simulink model "position_control_2015"  (R2020a)
settings: Solver=ode4  StartTime=0.0  StopTime=inf  FixedStep=0.002  RelTol=1e-3  EnableMultiTasking=on
undefined symbols (not defined in the file): Afe, g, gain_stab9, gains_increasing, I_eq_increasing, K, Kp_i_increasing, Kp_mf_increasing, L, m, m0, REG_m9_f, Ti_i_increasing, Ti_mf_increasing, x, x_eq, x_eq_increasing, y
libraries: simulink x8, PoliArd x6
settings Model: ExtModeTrigDuration=2  Creator=User  LastModifiedBy=miche
settings DataIOCC: LimitDataPoints=on  SaveFormat=Array  ReturnWorkspaceOutputs=off
settings OptimizationCC: LifeSpan=1  EfficientTunableParamExpr=on
settings DebuggingCC: UnderspecifiedInitializationDetection=Classic  MergeDetectMultiDrivingBlocksExec=none  SFUnexpectedBacktrackingDiag=warning  SFNoUnconditionalDefaultTransitionDiag=warning  SFExecutionAtInitializationDiag=none  ArithmeticOperatorsInVariantConditions=warning
settings HardwareCC: ProdBitPerPointer=32  ProdBitPerSizeT=32  ProdBitPerPtrDiffT=32  ProdLargestAtomicInteger=Long  ProdLargestAtomicFloat=Double  ProdIntDivRoundTo=Undefined  ProdWordSize=32  ProdHWDeviceType=ARM Compatible->ARM Cortex
settings ModelReferenceCC: PropagateSignalLabelsOutOfModel=off
settings SFSimCC: SimUseLocalCustomCode=off  MATLABDynamicMemAlloc=off  CustomCodeUndefinedFunction=UseInterfaceOnly
settings RTWCC: Description=Run on Target Hardware  SystemTargetFile=realtime.tlc  GenerateMakefile=off  TemplateMakefile=realtime.tmf  RTWVerbose=off  RTWUseLocalCustomCode=off
settings CodeAppCC: StateflowObjectComments=on
settings STFCustomTargetCC: TargetLibSuffix=.a  GenerateSampleERTMain=on  ERTCustomFileBanners=on  SupportNonInlinedSFcns=off  RemoveResetFunc=on  SupportVariableSizeSignals=on  MATLABClassNameForMDSCustomization=Simulink.SoftwareTarget.ERTCustomization  SystemTargetFile=realtime.tlc
settings ERTTargetCC: MultiwordLength=2048  GenerateSampleERTMain=on  ParMdlRefBuildCompliant=off  CompOptLevelCompliant=off  ConcurrentExecutionCompliant=off  CombineOutputUpdateFcns=off  SupportContinuousTime=on  SupportVariableSizeSignals=on  ModelStepFunctionPrototypeControlCompliant=off  CPPClassGenCompliant=off  UseToolchainInfoCompliant=off  ExtModeTransport=3  ExtModeMexFile=ext_serial_win32_comm_rtt  ExtModeMexArgs=0 1 9600  ERTSrcFileBannerTemplate=realtime_code_template.cgt  ERTHdrFileBannerTemplate=realtime_code_template.cgt  ERTDataSrcFileTemplate=realtime_code_template.cgt  ERTDataHdrFileTemplate=realtime_code_template.cgt  ERTCustomFileTemplate=realtime_file_process.tlc  ConvertIfToSwitch=off  SuppressUnreachableDefaultCases=off
settings ConfigComp: CovMetricSettings=dw  CovSaveCumulativeToWorkspaceVar=on  CovSaveSingleToWorkspaceVar=on  CovExternalEMLEnable=off

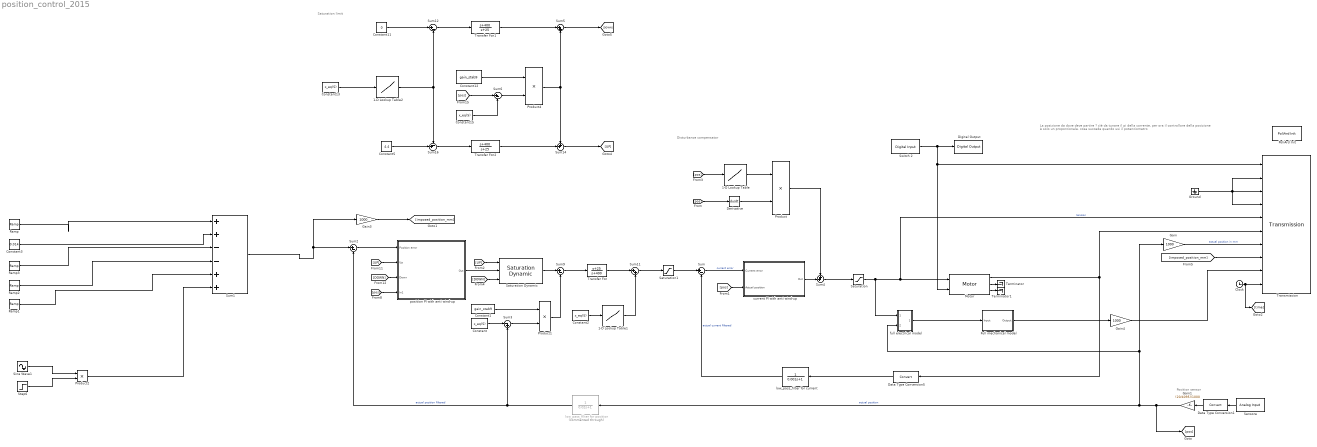
== system position_control_2015 ==
  note: Saturation limit
  note: Position sensor
  note: Disturbance compensator
  note: La posizione da dove deve partire ? cìè da tunare il pi della corrente, per ora il controllore della posizione è solo un
      | proporzionale. cosa succede quando usi il potenziometro
  1-D Lookup Table : Lookup_n-D  NumberOfTableDimensions=1  BreakpointsForDimension1=[0.0085 x_eq_increasing]  Table=[gains_increasing(1) gains_increasing]  InternalRulePriority=Speed  RndMeth=Simplest  InputSameDT=on
  1-D Lookup Table1 : Lookup_n-D  NumberOfTableDimensions=1  BreakpointsForDimension1=[0.0085 x_eq_increasing]  Table=[3.55 I_eq_increasing]  InternalRulePriority=Speed  RndMeth=Simplest  InputSameDT=on
  1-D Lookup Table2 : Lookup_n-D  NumberOfTableDimensions=1  BreakpointsForDimension1=[0.0085 x_eq_increasing]  Table="[3.55  I_eq_increasing]"  InternalRulePriority=Speed  RndMeth=Simplest  InputSameDT=on
  Clock : Clock
  Constant{,2,13,15} (4 alike) : Constant  Value=x_eq(5)
  Constant1 : Constant  Value=gain_stab9
  Constant11 : Constant  Value=0
  Constant12 : Constant  Value=gain_stab9
  Constant3 : Constant  Value=0.014
  Constant5 : Constant  Value=4.4
  Data Type Conversion1 : DataTypeConversion
  Data Type Conversion5 : DataTypeConversion
  Derivative : Derivative
  Digital Output : PoliArd/Digital Output  DO_pin=1
  Full mechanical model : Subsystem
  Gain : Gain  Gain=1000
  Gain1 : Gain  Gain=(20/4095)/1000
  Gain3 : Gain  Gain=1000
  Gain4 : Gain  Gain=1000
  Ground : Ground
  Motor : PoliArd/Motor  MotorID=2  DC_bus_mask=24  dt_mot=-1
  PoliArd Init : PoliArd/PoliArd Init
  Product{,1..2,4} (4 alike) : Product
  Ramp : simulink/Sources/Ramp  slope=0.001  start=7  InitialOutput=0
  Ramp1 : simulink/Sources/Ramp  slope=0.001  start=19  InitialOutput=0
  Ramp2 : simulink/Sources/Ramp  slope=0.001  start=17  InitialOutput=0
  Ramp3 : simulink/Sources/Ramp  slope=0.001  start=12  InitialOutput=0
  Saturation : Saturate  UpperLimit=18  LowerLimit=0
  Saturation Dynamic : simulink/Discontinuities/Saturation Dynamic  OutMin=[]  OutMax=[]  OutDataTypeStr=Inherit: Same as second input  OutDataType=fixdt(1, 16)  OutScaling=2^-10  DoSatur=off
  Saturation1 : Saturate  UpperLimit=4.4  LowerLimit=0
  Sensore : PoliArd/Analog Input  AIpin_mask=2  AIsample=-1
  Sine Wave1 : Sin  Amplitude=0.002  Phase=0.3  SampleTime=0
  Step6 : Step  Time=28  SampleTime=0
  Sum{,2,6,9,12} (5 alike) : Sum  Inputs=|+-
  Sum1 : Sum  Inputs=|++--++
  Sum11 : Sum  Inputs=|++
  Sum14 : Sum  Inputs=++|
  Sum16 : Sum  Inputs=-+|
  Sum3 : Sum  Inputs=|-+
  Sum4 : Sum  Inputs=++|
  Sum5 : Sum  Inputs=|++
  Switch 2 : PoliArd/Digital Input  DI_pin=2  DIsample=-1
  Terminator : Terminator
  Terminator1 : Terminator
  Transfer Fcn : TransferFcn  Numerator=[1 25]  Denominator=[1 400]
  Transfer Fcn1 : TransferFcn  Numerator=[1 400]  Denominator=[1 25]
  Transfer Fcn2 : TransferFcn  Numerator=[1 400]  Denominator=[1 25]
  Transmission : PoliArd/Transmission  sample_freq=500  sig_to_send=6
  current PI with anti wind-up : Subsystem
      mask Display: disp('Current controller\n(PI)\nwith anti wind-up')
  full electrical model : Subsystem
  low_pass_filter for current : TransferFcn  Denominator=[0.001 1]
  low_pass_filter for position : TransferFcn  Commented=through  Denominator=[0.02 1]
  position PI with anti wind-up : Subsystem
      mask Display: disp('Position controller\n(PI)\nwith anti wind-up')
  wires:
  Switch 2/1 -> Digital Output/1, Motor/2, Transmission/1
  Sensore/1 -> Data Type Conversion1/1
  Ground/1 -> Transmission/2, Transmission/4, Transmission/3
  Motor/1 -> Data Type Conversion5/1, Transmission/6
  Data Type Conversion1/1 -> Gain1/1
  Saturation/1 -> full electrical model/1(In1), Transmission/5, Motor/1  "tension"
  Constant1/1 -> Product1/1
  Sum9/1 -> Transfer Fcn/1
  Sum11/1 -> Saturation1/1
  [DOWN] -> Saturation Dynamic/3
  1-D Lookup Table1/1 -> Sum11/2
  Product/1 -> Sum4/1
  Saturation Dynamic/1 -> Sum9/1
  Derivative/1 -> Product/2
  Sum2/1 -> position PI with anti wind-up/1(Position error)
  1-D Lookup Table/1 -> Product/1
  current PI with anti wind-up/1(Out) -> Sum4/2
  Sum/1 -> current PI with anti wind-up/1(Current error)  "current error"
  position PI with anti wind-up/1(Out) -> Saturation Dynamic/2
  [pos] -> 1-D Lookup Table/1
  Sum3/1 -> Product1/2
  Product1/1 -> Sum9/2
  [UP] -> Saturation Dynamic/1
  Transfer Fcn/1 -> Sum11/1
  [pos] -> current PI with anti wind-up/2(Actual position)
  Sum4/1 -> Saturation/1
  Saturation1/1 -> Sum/1
  [pos] -> Derivative/1
  Data Type Conversion5/1 -> low_pass_filter for current/1
  Gain1/1 -> full electrical model/2(In2), Gain/1, low_pass_filter for position/1, [pos]  "actual position"
  low_pass_filter for current/1 -> Sum/2  "actual current filtered"
  low_pass_filter for position/1 -> Sum2/2, Sum3/2  "actual position filtered"
  Constant2/1 -> 1-D Lookup Table1/1
  Gain/1 -> Transmission/7  "actual position in mm"
  [DOWN] -> position PI with anti wind-up/3(Down)
  [UP] -> position PI with anti wind-up/2(Up)
  [imposed_position_mm] -> Transmission/8
  Motor/2 -> Terminator/1
  Motor/3 -> Terminator1/1
  Constant/1 -> Sum3/1
  Sum5/1 -> [DOWN]
  Constant15/1 -> Sum6/2
  Sum12/1 -> Transfer Fcn1/1
  Product4/1 -> Sum14/1, Sum5/2
  1-D Lookup Table2/1 -> Sum16/1, Sum12/2
  Sum16/1 -> Transfer Fcn2/1
  Sum6/1 -> Product4/2
  Constant13/1 -> 1-D Lookup Table2/1
  Constant11/1 -> Sum12/1
  [pos] -> Sum6/1
  Transfer Fcn2/1 -> Sum14/2
  Sum14/1 -> [UP]
  Transfer Fcn1/1 -> Sum5/1
  Constant12/1 -> Product4/1
  Constant5/1 -> Sum16/2
  [pos] -> position PI with anti wind-up/4(In1)
  Gain3/1 -> [imposed_position_mm]
  Clock/1 -> Transmission/10, [time]
  Ramp/1 -> Sum1/1
  Constant3/1 -> Sum1/2
  Ramp3/1 -> Sum1/3
  Ramp2/1 -> Sum1/4
  Ramp1/1 -> Sum1/5
  Sine Wave1/1 -> Product2/1
  Step6/1 -> Product2/2
  Product2/1 -> Sum1/6
  Sum1/1 -> Gain3/1, Sum2/1
  full electrical model/1(Input) -> Full mechanical model/1(Input)
  Full mechanical model/1(Output) -> Gain4/1
  Gain4/1 -> Transmission/9

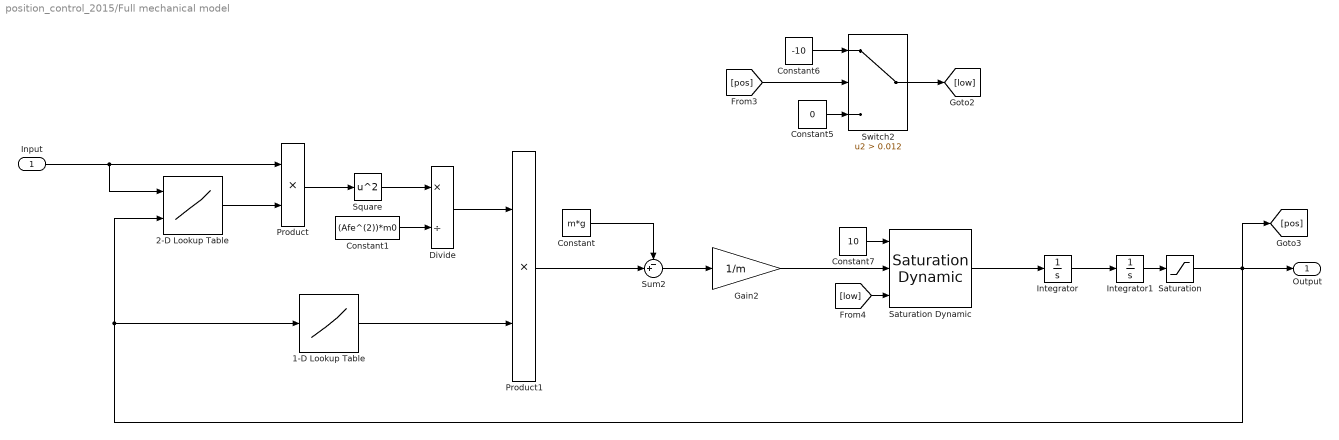
== system position_control_2015/Full mechanical model ==
  Input : Inport
  1-D Lookup Table : Lookup_n-D  NumberOfTableDimensions=1  BreakpointsForDimension1=x  Table=K  InternalRulePriority=Speed  RndMeth=Simplest  InputSameDT=on
  2-D Lookup Table : Lookup_n-D  BreakpointsForDimension1=y  BreakpointsForDimension2=x  Table=L  InternalRulePriority=Speed  RndMeth=Simplest  InputSameDT=on
  Constant : Constant  Value=m*g
  Constant1 : Constant  Value=(Afe^(2))*m0
  Constant5 : Constant  Value=0
  Constant6 : Constant  Value=-10
  Constant7 : Constant  Value=10
  Divide : Product  Inputs=*/
  Gain2 : Gain  Gain=1/m
  Integrator : Integrator
  Integrator1 : Integrator  InitialCondition=0.0085
  Product : Product
  Product1 : Product
  Saturation : Saturate  UpperLimit=0.020  LowerLimit=0.0085
  Saturation Dynamic : simulink/Discontinuities/Saturation Dynamic  OutMin=[]  OutMax=[]  OutDataTypeStr=Inherit: Same as second input  OutDataType=fixdt(1, 16)  OutScaling=2^-10  DoSatur=off
  Square : Math  Operator=square  SignedPower=on  SaturateOnIntegerOverflow=on
  Sum2 : Sum  Inputs=-+|
  Switch2 : Switch  Criteria=u2 > Threshold  Threshold=0.012
  Output : Outport
  wires:
  Input/1 -> Product/1, 2-D Lookup Table/1
  Square/1 -> Divide/1
  Constant/1 -> Sum2/1
  Product1/1 -> Sum2/2
  Product/1 -> Square/1
  Constant1/1 -> Divide/2
  2-D Lookup Table/1 -> Product/2
  Divide/1 -> Product1/1
  1-D Lookup Table/1 -> Product1/2
  Integrator1/1 -> Saturation/1
  Integrator/1 -> Integrator1/1
  Sum2/1 -> Gain2/1
  Constant6/1 -> Switch2/1
  [pos] -> Switch2/2
  Switch2/1 -> [low]
  Constant5/1 -> Switch2/3
  [low] -> Saturation Dynamic/3
  Constant7/1 -> Saturation Dynamic/1
  Saturation/1 -> 1-D Lookup Table/1, 2-D Lookup Table/2, Output/1, [pos]
  Gain2/1 -> Saturation Dynamic/2
  Saturation Dynamic/1 -> Integrator/1

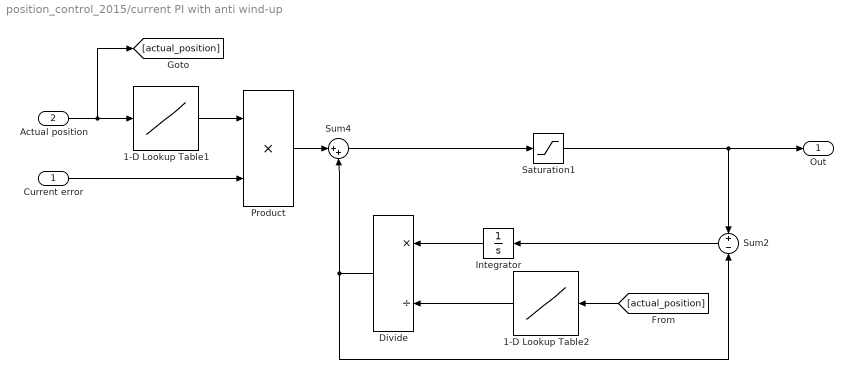
== system position_control_2015/current PI with anti wind-up ==
  Current error : Inport
  Actual position : Inport  Port=2
  1-D Lookup Table1 : Lookup_n-D  NumberOfTableDimensions=1  BreakpointsForDimension1=[0.0085 x_eq_increasing]  Table=[Kp_i_increasing(1) Kp_i_increasing]  InternalRulePriority=Speed  RndMeth=Simplest  InputSameDT=on
  1-D Lookup Table2 : Lookup_n-D  NumberOfTableDimensions=1  BreakpointsForDimension1=[0.0085 x_eq_increasing]  Table=[Ti_i_increasing(1) Ti_i_increasing]  InternalRulePriority=Speed  RndMeth=Simplest  InputSameDT=on
  Divide : Product  Inputs=*/
  Integrator : Integrator
  Product : Product
  Saturation1 : Saturate  UpperLimit=18  LowerLimit=0
  Sum2 : Sum  Inputs=+|-
  Sum4 : Sum  Inputs=|++
  Out : Outport
  wires:
  Sum4/1 -> Saturation1/1
  Product/1 -> Sum4/1
  Saturation1/1 -> Out/1, Sum2/1
  Current error/1 -> Product/2
  1-D Lookup Table1/1 -> Product/1
  Actual position/1 -> [actual_position], 1-D Lookup Table1/1
  Divide/1 -> Sum2/2, Sum4/2
  Sum2/1 -> Integrator/1
  Integrator/1 -> Divide/1
  1-D Lookup Table2/1 -> Divide/2
  [actual_position] -> 1-D Lookup Table2/1

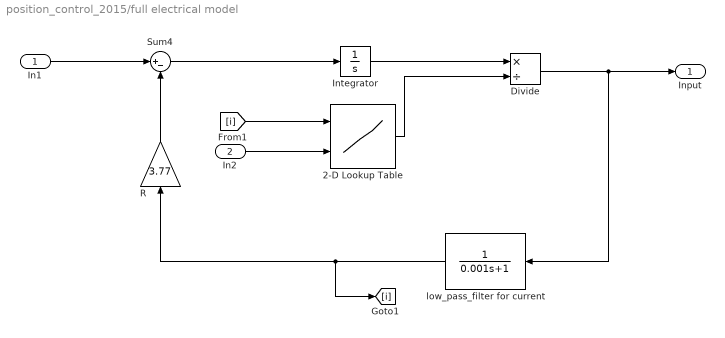
== system position_control_2015/full electrical model ==
  In1 : Inport
  In2 : Inport  Port=2
  2-D Lookup Table : Lookup_n-D  BreakpointsForDimension1=y  BreakpointsForDimension2=x  Table=L  InternalRulePriority=Speed  RndMeth=Simplest  InputSameDT=on
  Divide : Product  Inputs=*/
  Integrator : Integrator
  R : Gain  Gain=3.77
  Sum4 : Sum  Inputs=|+-
  low_pass_filter for current : TransferFcn  Denominator=[0.001 1]
  Input : Outport
  wires:
  Sum4/1 -> Integrator/1
  Integrator/1 -> Divide/1
  R/1 -> Sum4/2
  In2/1 -> 2-D Lookup Table/2
  2-D Lookup Table/1 -> Divide/2
  In1/1 -> Sum4/1
  [i] -> 2-D Lookup Table/1
  Divide/1 -> low_pass_filter for current/1, Input/1
  low_pass_filter for current/1 -> [i], R/1

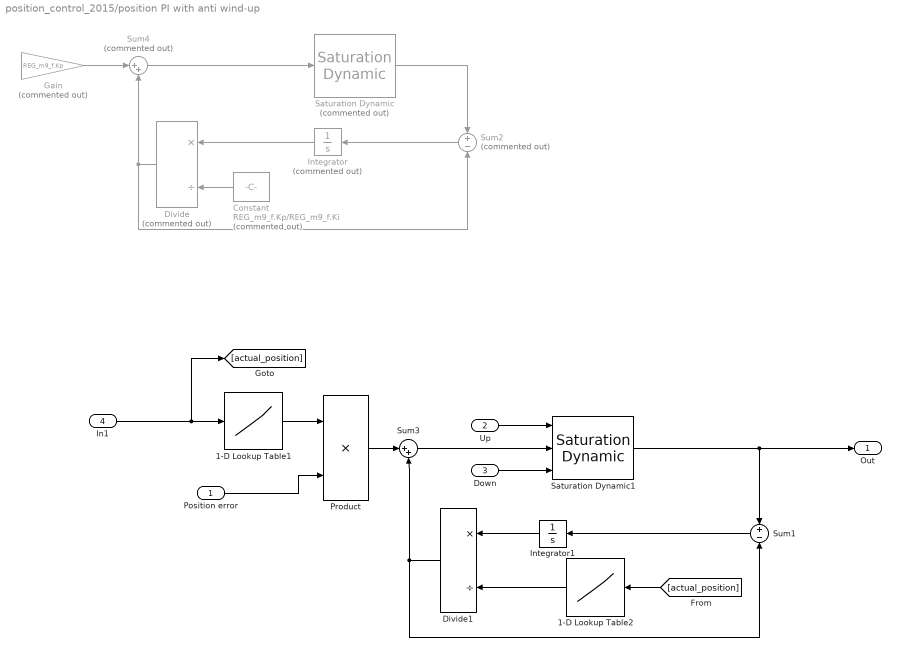
== system position_control_2015/position PI with anti wind-up ==
  Position error : Inport
  Up : Inport  Port=2
  Down : Inport  Port=3
  In1 : Inport  Port=4
  1-D Lookup Table1 : Lookup_n-D  NumberOfTableDimensions=1  BreakpointsForDimension1=[0.0085 x_eq_increasing]  Table=[Kp_mf_increasing(1) Kp_mf_increasing]  InternalRulePriority=Speed  RndMeth=Simplest  InputSameDT=on
  1-D Lookup Table2 : Lookup_n-D  NumberOfTableDimensions=1  BreakpointsForDimension1=[0.0085 x_eq_increasing]  Table=[Ti_mf_increasing(1) Ti_mf_increasing]  InternalRulePriority=Speed  RndMeth=Simplest  InputSameDT=on
  Constant : Constant  Commented=on  Value=REG_m9_f.Kp/REG_m9_f.Ki
  Divide : Product  Commented=on  Inputs=*/
  Divide1 : Product  Inputs=*/
  Gain : Gain  Commented=on  Gain=REG_m9_f.Kp
  Integrator : Integrator  Commented=on
  Integrator1 : Integrator
  Product : Product
  Saturation Dynamic : simulink/Discontinuities/Saturation Dynamic  Commented=on  OutMin=[]  OutMax=[]  OutDataTypeStr=Inherit: Same as second input  OutDataType=fixdt(1, 16)  OutScaling=2^-10  DoSatur=off
  Saturation Dynamic1 : simulink/Discontinuities/Saturation Dynamic  OutMin=[]  OutMax=[]  OutDataTypeStr=Inherit: Same as second input  OutDataType=fixdt(1, 16)  OutScaling=2^-10  DoSatur=off
  Sum1 : Sum  Inputs=+|-
  Sum2 : Sum  Commented=on  Inputs=+|-
  Sum3 : Sum  Inputs=|++
  Sum4 : Sum  Commented=on  Inputs=|++
  Out : Outport
  wires:
  Gain/1 -> Sum4/1
  Constant/1 -> Divide/2
  Sum2/1 -> Integrator/1
  Divide/1 -> Sum2/2, Sum4/2
  Integrator/1 -> Divide/1
  Sum4/1 -> Saturation Dynamic/2
  Saturation Dynamic/1 -> Sum2/1
  [actual_position] -> 1-D Lookup Table2/1
  Divide1/1 -> Sum1/2, Sum3/2
  1-D Lookup Table2/1 -> Divide1/2
  Integrator1/1 -> Divide1/1
  Sum1/1 -> Integrator1/1
  1-D Lookup Table1/1 -> Product/1
  Saturation Dynamic1/1 -> Out/1, Sum1/1
  Product/1 -> Sum3/1
  Sum3/1 -> Saturation Dynamic1/2
  Position error/1 -> Product/2
  In1/1 -> [actual_position], 1-D Lookup Table1/1
  Up/1 -> Saturation Dynamic1/1
  Down/1 -> Saturation Dynamic1/3
